simulink model "ModelLTI"  (R2013b)
settings: Solver=ode45  StartTime=0.0  StopTime=10.0  RelTol=1e-3
values from neighbouring files (symbols this model uses):
  D = xopt(3)    [Plant1delay.m]    (also in Plant2.m; Plant2delay.m; Plant3.m; Plant4.m)
  I = xopt(2)    [Plant1delay.m]    (also in Plant2.m; Plant2delay.m; Plant3.m; Plant4.m)
  N = xopt(4)    [Plant1delay.m]    (also in Plant2.m; Plant2delay.m; Plant3.m; Plant4.m)
  P = xopt(1)    [Plant1delay.m]    (also in Plant2.m; Plant2delay.m; Plant3.m; Plant4.m)
libraries: simulink x2, cstblocks x1
settings Model: Creator=stelmo  LastModifiedBy=stelmo

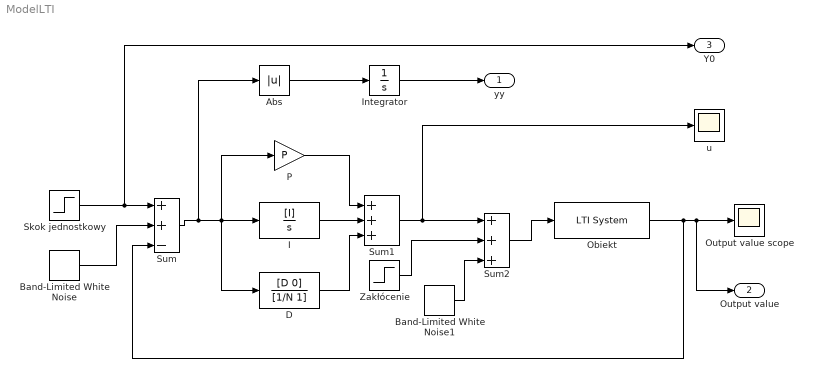
== system ModelLTI ==
  Abs : Abs
  Band-Limited White Noise : simulink/Sources/Band-Limited White Noise  Cov=[0.000001]  Ts=0.01  seed=[23341]
  Band-Limited White Noise1 : simulink/Sources/Band-Limited White Noise  Cov=[0.000001]  Ts=0.01  seed=[23341]
  D : TransferFcn  Numerator=[D 0]  Denominator=[1/N 1]
  I : TransferFcn  Numerator=[I]  Denominator=[1 0]
  Integrator : Integrator
  Obiekt : cstblocks/LTI System  sys=G  IC=[]
  Output value scope : Scope
      settings: MaxDataPoints=50000000
  P : Gain  Gain=P
  Skok jednostkowy : Step  SampleTime=0
  Sum : Sum  Inputs=++-
  Sum1 : Sum  Inputs=+++
  Sum2 : Sum  Inputs=+++
  Zakłócenie : Step  SampleTime=0
  u : Scope
  yy : Outport
  Output value : Outport  Port=2
  Y0 : Outport  Port=3
  wires:
  Obiekt/1 -> Sum/3, Output value/1, Output value scope/1
  Abs/1 -> Integrator/1
  Integrator/1 -> yy/1
  P/1 -> Sum1/1
  I/1 -> Sum1/2
  D/1 -> Sum1/3
  Sum/1 -> Abs/1, D/1, P/1, I/1
  Skok jednostkowy/1 -> Y0/1, Sum/1
  Sum1/1 -> u/1, Sum2/1
  Sum2/1 -> Obiekt/1
  Zakłócenie/1 -> Sum2/2
  Band-Limited White Noise/1 -> Sum/2
  Band-Limited White Noise1/1 -> Sum2/3
